simulink model "SensoryAttenuationTask"  (R2019b)
settings: Solver=ode4  StartTime=0.0  StopTime=inf  FixedStep=BKIN_STEP_TIME  RelTol=1e-3  EnableMultiTasking=on
StartFcn:
  |  warndlg('Dexterit-E models cannot run under simulation. Please compile your model and run it from within Dexterit-E.');set_param(bdroot,'SimulationCommand','stop')
model workspace (MAT data in the model file):
  BKIN_KINEMATIC_FRAME_SIZE = 400
  BKIN_STEP_TIME = 0.00025
  COLOR_2ND = 5
  COLOR_INIT = 4
  EDGE_COLOUR = 8
  EDGE_WIDTH = 9
  E_HAND_IN_START = 2
  E_MATCH_CHECK_ON = 8
  E_MATCH_END = 9
  E_MATCH_ON = 7
  E_MATCH_START = 8
  E_NO_EVENT = 0
  E_SLIDER_CHECK_ON = 4
  E_SLIDER_END = 5
  E_SLIDER_START = 10
  E_TEST_FORCE_ON = 3
  E_TIMED_OUT = 11
  E_TRIAL_END = 6
  E_TRIAL_START = 1
  HOLD_DELAY = 3
  LEFT_COL = 1
  LENGTH = 6
  LOAD_COL = 9
  LOAD_TIME = 4
  LOAD_X = 1
  LOAD_Y = 2
  MATCH_COL = 5
  MATCH_C_COL = 6
  MATCH_SCALING = 8
  MAX_START_TIME = 1
  RADIUS_VIS = 3
  RAMP_DURATION = 5
  RAMP_DURATION_EXAM = 6
  RIGHT_COL = 2
  SAFETY_DIST = 12
  SAFETY_SCALING = 13
  SLIDER_COL = 3
  SLIDER_C_COL = 4
  SLIDER_SCALING = 7
  SLOW_THRESH = 11
  TEXT = 10
  TEXT2_COL = 8
  TEXT_COL = 7
  TEXT_DISTH = 10
  TEXT_DISTV = 9
  TEXT_SIZE = 11
  WIDTH = 7
  WITHIN_DELAY = 2
  col_x = 1
  col_y = 2
undefined symbols (not defined in the file): slselsubs
libraries: Video x9, KINARM_general x5, General x3, KINARM_EP_loads x3
settings Model: ModifiedComment=chris -- Wed Feb 16 09:18:30 2005 -- Version 1.1384  ModifiedHistory=Feb 16/05 - Add error repeat, add offset ramp  ExtModeArmWhenConnect=off  ExtModeLogAll=off  OrderedModelArguments=off  Creator=Chris Grebeldinger  LastModifiedBy=User
settings SolverCC: AutoInsertRateTranBlk=on
settings DataIOCC: SaveFormat=Array  SignalLoggingSaveFormat=ModelDataLogs  SaveOutput=off  SaveTime=off  ReturnWorkspaceOutputs=off  SignalLoggingName=sigsOut
settings OptimizationCC: BlockReduction=off  BooleanDataType=off  OptimizeBlockIOStorage=off  BufferReuse=off  GlobalBufferReuse=off  ExpressionFolding=off  ExpressionDepthLimit=2147483647  LocalBlockOutputs=off  InitFltsAndDblsToZero=on  LifeSpan=inf  OptimizeDataStoreBuffers=off  BusAssignmentInplaceUpdate=off
settings DebuggingCC: SaveWithParameterizedLinksMsg=none  UnderspecifiedInitializationDetection=Classic  MergeDetectMultiDrivingBlocksExec=none  SignalResolutionControl=TryResolveAllWithWarning  MultiTaskDSMMsg=warning  FcnCallInpInsideContextMsg=warning  BusObjectLabelMismatch=none  StateNameClashWarn=warning  StrictBusMsg=ErrorOnBusTreatedAsVector  SFUnexpectedBacktrackingDiag=warning  SFNoUnconditionalDefaultTransitionDiag=warning  SFExecutionAtInitializationDiag=none  UnderSpecifiedDimensionMsg=warning  ArithmeticOperatorsInVariantConditions=warning
settings HardwareCC: ProdBitPerPointer=32  ProdBitPerSizeT=32  ProdBitPerPtrDiffT=32  ProdLargestAtomicFloat=None  ProdWordSize=32  ProdLongLongMode=on  ProdHWDeviceType=Generic->32-bit x86 compatible  TargetLongLongMode=on  TargetIntDivRoundTo=Zero  TargetEndianess=LittleEndian  TargetHWDeviceType=Generic->32-bit x86 compatible
settings ModelReferenceCC: PropagateSignalLabelsOutOfModel=off
settings SFSimCC: SimCustomHeaderCode="#include \"stdlib.h\""  SimUseLocalCustomCode=off  SimParseCustomCode=off  CustomCodeUndefinedFunction=UseInterfaceOnly
settings RTWCC: Description=Simulink Real-Time  SystemTargetFile=slrt.tlc  TemplateMakefile=slrt_default_tmf  RTWUseLocalCustomCode=off  CustomSourceCode="#include \"stdlib.h\""  CodeExecutionProfiling=on
settings CodeAppCC: MaxIdLength=63  StateflowObjectComments=on
settings SimulinkRealTimeCC: TargetFcnLib=ansi_tfl_tmw.mat  GeneratePreprocessorConditionals=Disable all  PreserveStateflowLocalDataDimensions=off
settings ConfigComp: CovMetricSettings=dw  CovHtmlReporting=on  CovSaveCumulativeToWorkspaceVar=on  CovSaveSingleToWorkspaceVar=on  CovExternalEMLEnable=off

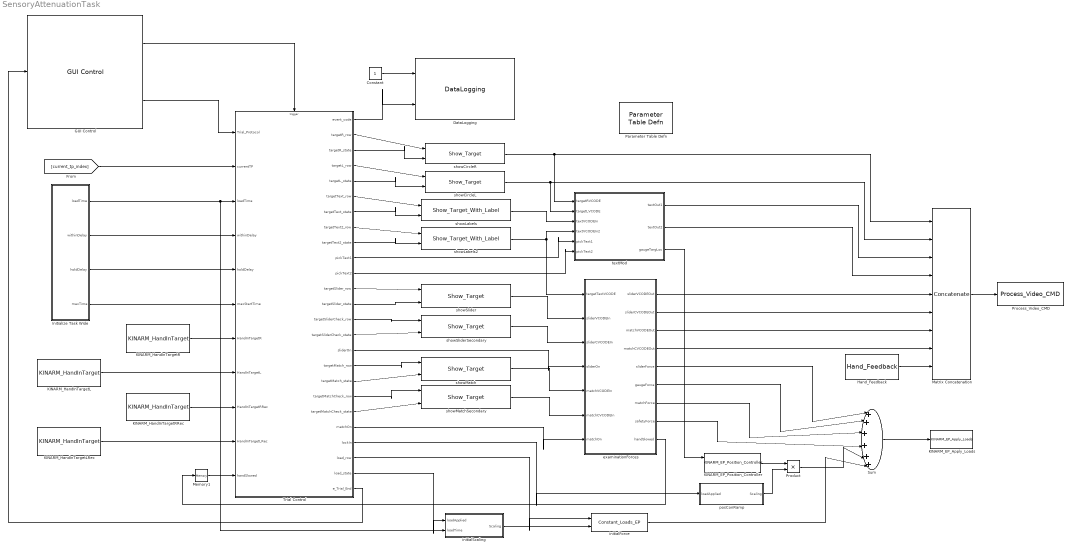
== system SensoryAttenuationTask ==
  Constant : Constant
  DataLogging : General/DataLogging  log_event_codes=on  log_analog_inputs=off  show_time_remaining=off  ecat_include=on
  GUI Control : General/GUI Control  task_version=1.0  show_repeat_trial_flag=off  use_custom_tp=off  target_type_str=Circle  Target_Type=1  XYcols=[1 2]  Vcols=3  Lcols=4  indices_padding=[0 0 0 0;0 0 0 0]  target_table_rows=64  load_table_rows=20  tp_table_rows=100
  Hand_Feedback : KINARM_general/Hand_Feedback  feedback_cntl_src=none
  Initialize Task Wide : Subsystem
  KINARM_EP_Apply_Loads : KINARM_EP_loads/KINARM_EP_Apply_Loads  up_duration=1500  down_duration=1500  max_force=15
  KINARM_EP_Position_Controller : KINARM_EP_loads/KINARM_EP_Position_Controller  use_dom_hand=off  inertias_for_FF=KINARM End Point robot  gain_choice=Standard Movement  sample_time=0.001
  KINARM_HandInTargetL : KINARM_general/KINARM_HandInTarget  use_dominant_hand=off  target_type=Circle  num_states=1  attribcol1=[RADIUS_VIS]  attribcol2=[0]  attribcol3=[0]  attribcol4=[0]  attribcol5=[0]
  KINARM_HandInTargetLRec : KINARM_general/KINARM_HandInTarget  use_dominant_hand=off  target_type=Rectangle  num_states=1  attribcol1=[WIDTH LENGTH 0]  attribcol2=[0 0 0]  attribcol3=[0 0 0]  attribcol4=[0 0 0]  attribcol5=[0 0 0]
  KINARM_HandInTargetR : KINARM_general/KINARM_HandInTarget  use_dominant_hand=on  target_type=Circle  num_states=1  attribcol1=[RADIUS_VIS]  attribcol2=[0]  attribcol3=[0]  attribcol4=[0]  attribcol5=[0]
  KINARM_HandInTargetRRec : KINARM_general/KINARM_HandInTarget  use_dominant_hand=on  target_type=Rectangle  num_states=1  attribcol1=[WIDTH LENGTH 0]  attribcol2=[0 0 0]  attribcol3=[0 0 0]  attribcol4=[0 0 0]  attribcol5=[0 0 0]
  Matrix Concatenation : Concatenate  NumInputs=9  Mode=Multidimensional array
  Memory1 : Memory
  Parameter Table Defn : General/Parameter Table Defn  ShowInLibBrowser=0
  Process_Video_CMD : Video/Process_Video_CMD  video_delay=50
  Product : Product
  Sum : Sum  Inputs=|++++++|
  Trial Control : Stateflow chart  TreatAsAtomicUnit=on
  examinationForces : Subsystem
  initialForce : KINARM_EP_loads/Constant_Loads_EP  use_dom_hand=on  loadcol=[1 2]  source=port  scaling=1  use_LH_coord=on
  initialScaling : Subsystem  mask(Perturbation){}
  posConRamp : Subsystem  mask(Perturbation){}
  showCircleL : Video/Show_Target  target_type=Circle  num_states=1  attribcol1=[COLOR_INIT 0 0 RADIUS_VIS]  attribcol2=[0 0 0 0]  attribcol3=[0 0 0 0]  attribcol4=[0 0 0 0]  attribcol5=[0 0 0 0]  stateindices_padding=[0 0 0 0 0 0 0;0 0 0 0 0 0 0;0 0 0 0 0 0 0;0 0 0 0 0 0 0;0 0 0 0 0 0 0]  source=dialog  opacity=100  target_display=Both subject and operator displays  num_col=4
  showCircleR : Video/Show_Target  target_type=Circle  num_states=1  attribcol1=[COLOR_INIT 0 0 RADIUS_VIS]  attribcol2=[0 0 0 0]  attribcol3=[0 0 0 0]  attribcol4=[0 0 0 0]  attribcol5=[0 0 0 0]  stateindices_padding=[0 0 0 0 0 0 0;0 0 0 0 0 0 0;0 0 0 0 0 0 0;0 0 0 0 0 0 0;0 0 0 0 0 0 0]  source=dialog  opacity=100  target_display=Both subject and operator displays  num_col=4
  showLabels : Video/Show_Target_With_Label  target_type=Circle  num_states=2  attribcol1=[0 0 0 0 TEXT COLOR_INIT TEXT_SIZE]  attribcol2=[0 0 0 0 TEXT COLOR_2ND RADIUS_VIS]  attribcol3=[0 0 0 0 0 0 0]  attribcol4=[0 0 0 0 0 0 0]  attribcol5=[0 0 0 0 0 0 0]  stateindices_padding=[0 0 0 0;0 0 0 0;0 0 0 0;0 0 0 0;0 0 0 0]  source=dialog  opacity=100  target_display=Both subject and operator displays
  showLabels2 : Video/Show_Target_With_Label  target_type=Circle  num_states=2  attribcol1=[0 0 0 0 TEXT COLOR_INIT TEXT_SIZE]  attribcol2=[0 0 0 0 TEXT COLOR_2ND RADIUS_VIS]  attribcol3=[0 0 0 0 0 0 0]  attribcol4=[0 0 0 0 0 0 0]  attribcol5=[0 0 0 0 0 0 0]  stateindices_padding=[0 0 0 0;0 0 0 0;0 0 0 0;0 0 0 0;0 0 0 0]  source=dialog  opacity=100  target_display=Both subject and operator displays
  showMatch : Video/Show_Target  target_type=Rectangle  num_states=1  attribcol1=[COLOR_INIT EDGE_COLOUR EDGE_WIDTH WIDTH LENGTH 0]  attribcol2=[0 0 0 0 0 0]  attribcol3=[0 0 0 0 0 0]  attribcol4=[0 0 0 0 0 0]  attribcol5=[0 0 0 0 0 0]  stateindices_padding=[0 0 0 0 0;0 0 0 0 0;0 0 0 0 0;0 0 0 0 0;0 0 0 0 0]  source=dialog  opacity=100  target_display=Both subject and operator displays  num_col=6
  showMatchSecondary : Video/Show_Target  target_type=Rectangle  num_states=2  attribcol1=[COLOR_INIT EDGE_COLOUR EDGE_WIDTH WIDTH LENGTH 0]  attribcol2=[COLOR_2ND EDGE_COLOUR EDGE_WIDTH WIDTH LENGTH 0]  attribcol3=[0 0 0 0 0 0]  attribcol4=[0 0 0 0 0 0]  attribcol5=[0 0 0 0 0 0]  stateindices_padding=[0 0 0 0 0;0 0 0 0 0;0 0 0 0 0;0 0 0 0 0;0 0 0 0 0]  source=dialog  opacity=100  target_display=Both subject and operator displays  num_col=6
  showSlider : Video/Show_Target  target_type=Rectangle  num_states=1  attribcol1=[COLOR_INIT EDGE_COLOUR EDGE_WIDTH WIDTH LENGTH 0]  attribcol2=[0 0 0 0 0 0]  attribcol3=[0 0 0 0 0 0]  attribcol4=[0 0 0 0 0 0]  attribcol5=[0 0 0 0 0 0]  stateindices_padding=[0 0 0 0 0;0 0 0 0 0;0 0 0 0 0;0 0 0 0 0;0 0 0 0 0]  source=dialog  opacity=100  target_display=Both subject and operator displays  num_col=6
  showSliderSecondary : Video/Show_Target  target_type=Rectangle  num_states=2  attribcol1=[COLOR_INIT COLOR_INIT EDGE_WIDTH WIDTH LENGTH 0]  attribcol2=[COLOR_2ND COLOR_2ND EDGE_WIDTH WIDTH LENGTH 0]  attribcol3=[0 0 0 0 0 0]  attribcol4=[0 0 0 0 0 0]  attribcol5=[0 0 0 0 0 0]  stateindices_padding=[0 0 0 0 0;0 0 0 0 0;0 0 0 0 0;0 0 0 0 0;0 0 0 0 0]  source=dialog  opacity=100  target_display=Both subject and operator displays  num_col=6
  textMod : Subsystem
  wires:
  Trial Control/25(e_Trial_End) -> GUI Control/1
  Trial Control/3(targetR_state) -> showCircleR/2
  Matrix Concatenation/1 -> Process_Video_CMD/1
  Trial Control/1(event_code) -> DataLogging/2
  showCircleR/1 -> textMod/1(targetRVCODE), Matrix Concatenation/1
  Hand_Feedback/1 -> Matrix Concatenation/9
  Constant/1 -> DataLogging/1
  GUI Control/2 -> Trial Control/1(Trial_Protocol)
  KINARM_HandInTargetR/1 -> Trial Control/7(HandInTargetR)
  KINARM_HandInTargetL/1 -> Trial Control/8(HandInTargetL)
  Initialize Task Wide/1(loadTime) -> initialScaling/2(loadTime), Trial Control/3(loadTime)
  Initialize Task Wide/2(withinDelay) -> Trial Control/4(withinDelay)
  Initialize Task Wide/4(maxTime) -> Trial Control/6(maxStartTime)
  [current_tp_index] -> Trial Control/2(currentTP)
  Trial Control/5(targetL_state) -> showCircleL/2
  Trial Control/14(targetSliderCheck_row) -> showSliderSecondary/1
  Trial Control/15(targetSliderCheck_state) -> showSliderSecondary/2
  Trial Control/24(load_state) -> initialScaling/1(loadApplied)
  initialScaling/1(Scaling) -> initialForce/2
  showSlider/1 -> examinationForces/2(sliderVCODEIn)
  showLabels/1 -> textMod/3(textVCODEIn)
  Trial Control/23(load_row) -> initialForce/1
  KINARM_HandInTargetRRec/1 -> Trial Control/9(HandInTargetRRec)
  KINARM_HandInTargetLRec/1 -> Trial Control/10(HandInTargetLRec)
  Trial Control/16(sliderOn) -> examinationForces/4(sliderOn)
  examinationForces/5(sliderForce) -> Sum/1
  initialForce/1 -> Sum/6
  Sum/1 -> KINARM_EP_Apply_Loads/1
  showMatch/1 -> examinationForces/5(matchVCODEIn)
  showMatchSecondary/1 -> examinationForces/6(matchCVCODEIn)
  Trial Control/19(targetMatchCheck_row) -> showMatchSecondary/1
  Trial Control/20(targetMatchCheck_state) -> showMatchSecondary/2
  examinationForces/7(matchForce) -> Sum/3
  examinationForces/6(gaugeForce) -> Sum/2
  Trial Control/21(matchOn) -> examinationForces/7(matchOn)
  Trial Control/10(pickText1) -> textMod/5(pickText1)
  Trial Control/11(pickText2) -> textMod/6(pickText2)
  textMod/2(textOut2) -> Matrix Concatenation/4
  textMod/1(textOut1) -> Matrix Concatenation/3
  Initialize Task Wide/3(holdDelay) -> Trial Control/5(holdDelay)
  Trial Control/12(targetSlider_row) -> showSlider/1
  Trial Control/17(targetMatch_row) -> showMatch/1
  Trial Control/18(targetMatch_state) -> showMatch/2
  Trial Control/13(targetSlider_state) -> showSlider/2
  Trial Control/2(targetR_row) -> showCircleR/1
  Trial Control/4(targetL_row) -> showCircleL/1
  showCircleL/1 -> textMod/2(targetLVCODE), Matrix Concatenation/2
  Trial Control/6(targetText_row) -> showLabels/1
  Trial Control/7(targetText_state) -> showLabels/2
  Trial Control/8(targetText2_row) -> showLabels2/1
  Trial Control/9(targetText2_state) -> showLabels2/2
  showLabels2/1 -> textMod/4(textVCODEIn2), examinationForces/1(targetTextVCODE)
  showSliderSecondary/1 -> examinationForces/3(sliderCVCODEIn)
  examinationForces/1(sliderVCODEOut) -> Matrix Concatenation/5
  examinationForces/2(sliderCVCODEOut) -> Matrix Concatenation/6
  examinationForces/3(matchVCODEOut) -> Matrix Concatenation/7
  GUI Control/1 -> Trial Control/Trigger
  Memory1/1 -> Trial Control/11(handSlowed)
  examinationForces/4(matchCVCODEOut) -> Matrix Concatenation/8
  textMod/3(gaugeTargLoc) -> KINARM_EP_Position_Controller/1
  KINARM_EP_Position_Controller/1 -> Product/1
  Product/1 -> Sum/5
  Trial Control/22(lockIn) -> posConRamp/1(loadApplied)
  posConRamp/1(Scaling) -> Product/2
  examinationForces/9(handSlowed) -> Memory1/1
  examinationForces/8(safetyForce) -> Sum/4

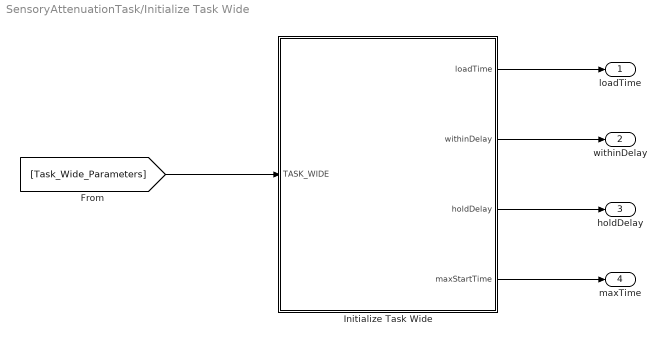
== system SensoryAttenuationTask/Initialize Task Wide ==
  Initialize Task Wide : MATLAB Function  TreatAsAtomicUnit=on
  loadTime : Outport
  withinDelay : Outport  Port=2
  holdDelay : Outport  Port=3
  maxTime : Outport  Port=4
  wires:
  [Task_Wide_Parameters] -> Initialize Task Wide/1(TASK_WIDE)
  Initialize Task Wide/1(loadTime) -> loadTime/1
  Initialize Task Wide/4(maxStartTime) -> maxTime/1
  Initialize Task Wide/2(withinDelay) -> withinDelay/1
  Initialize Task Wide/3(holdDelay) -> holdDelay/1

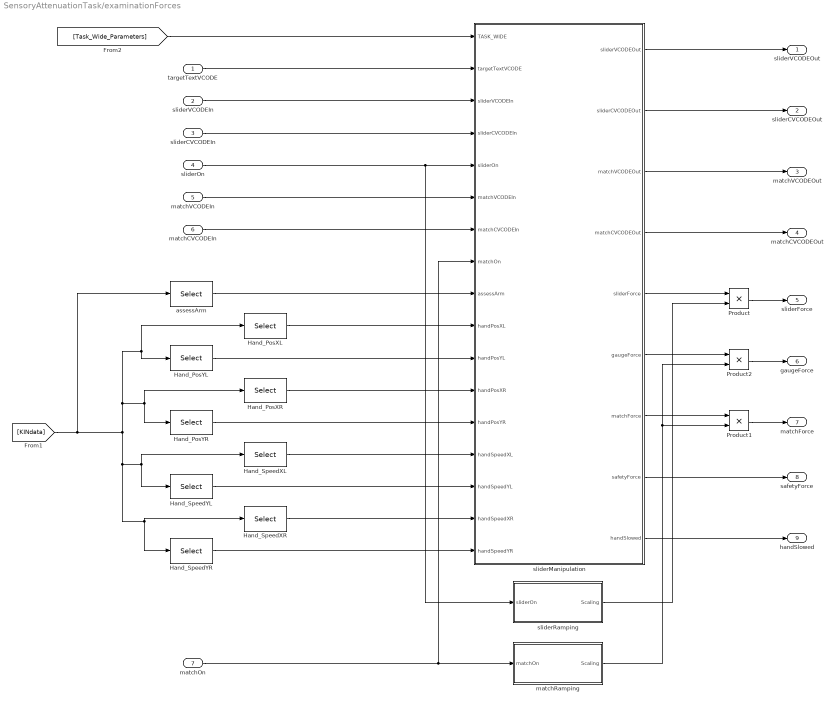
== system SensoryAttenuationTask/examinationForces ==
  targetTextVCODE : Inport
  sliderVCODEIn : Inport  Port=2
  sliderCVCODEIn : Inport  Port=3
  sliderOn : Inport  Port=4
  matchVCODEIn : Inport  Port=5
  matchCVCODEIn : Inport  Port=6
  matchOn : Inport  Port=7
  Hand_PosXL : Selector  NumberOfDimensions=2  InputPortWidth=3  IndexOptions=Index vector (dialog),Index vector (dialog)  Indices=[2],[23]  OutputSizes=slselsubs([(-2),(-2)],1),slselsubs([(-2),(-2)],2)
  Hand_PosXR : Selector  NumberOfDimensions=2  InputPortWidth=3  IndexOptions=Index vector (dialog),Index vector (dialog)  Indices=[1],[23]  OutputSizes=slselsubs([(-2),(-2)],1),slselsubs([(-2),(-2)],2)
  Hand_PosYL : Selector  NumberOfDimensions=2  InputPortWidth=3  IndexOptions=Index vector (dialog),Index vector (dialog)  Indices=[2],[24]  OutputSizes=slselsubs([(-2),(-2)],1),slselsubs([(-2),(-2)],2)
  Hand_PosYR : Selector  NumberOfDimensions=2  InputPortWidth=3  IndexOptions=Index vector (dialog),Index vector (dialog)  Indices=[1],[24]  OutputSizes=slselsubs([(-2),(-2)],1),slselsubs([(-2),(-2)],2)
  Hand_SpeedXL : Selector  NumberOfDimensions=2  InputPortWidth=3  IndexOptions=Index vector (dialog),Index vector (dialog)  Indices=[2],[25]  OutputSizes=slselsubs([(-2),(-2)],1),slselsubs([(-2),(-2)],2)
  Hand_SpeedXR : Selector  NumberOfDimensions=2  InputPortWidth=3  IndexOptions=Index vector (dialog),Index vector (dialog)  Indices=[1],[25]  OutputSizes=slselsubs([(-2),(-2)],1),slselsubs([(-2),(-2)],2)
  Hand_SpeedYL : Selector  NumberOfDimensions=2  InputPortWidth=3  IndexOptions=Index vector (dialog),Index vector (dialog)  Indices=[2],[26]  OutputSizes=slselsubs([(-2),(-2)],1),slselsubs([(-2),(-2)],2)
  Hand_SpeedYR : Selector  NumberOfDimensions=2  InputPortWidth=3  IndexOptions=Index vector (dialog),Index vector (dialog)  Indices=[1],[26]  OutputSizes=slselsubs([(-2),(-2)],1),slselsubs([(-2),(-2)],2)
  Product : Product
  Product1 : Product
  Product2 : Product
  assessArm : Selector  NumberOfDimensions=2  InputPortWidth=3  IndexOptions=Index vector (dialog),Index vector (dialog)  Indices=[3],[1]  OutputSizes=slselsubs([(-2),(-2)],1),slselsubs([(-2),(-2)],2)
  matchRamping : Subsystem  mask(Perturbation){}
  sliderManipulation : MATLAB Function  TreatAsAtomicUnit=on
  sliderRamping : Subsystem  mask(Perturbation){}
  sliderVCODEOut : Outport
  sliderCVCODEOut : Outport  Port=2
  matchVCODEOut : Outport  Port=3
  matchCVCODEOut : Outport  Port=4
  sliderForce : Outport  Port=5
  gaugeForce : Outport  Port=6
  matchForce : Outport  Port=7
  safetyForce : Outport  Port=8
  handSlowed : Outport  Port=9
  wires:
  sliderManipulation/2(sliderCVCODEOut) -> sliderCVCODEOut/1
  sliderManipulation/5(sliderForce) -> Product/1
  Hand_PosXR/1 -> sliderManipulation/12(handPosXR)
  Hand_PosXL/1 -> sliderManipulation/10(handPosXL)
  Hand_PosYL/1 -> sliderManipulation/11(handPosYL)
  Hand_PosYR/1 -> sliderManipulation/13(handPosYR)
  sliderCVCODEIn/1 -> sliderManipulation/4(sliderCVCODEIn)
  assessArm/1 -> sliderManipulation/9(assessArm)
  sliderVCODEIn/1 -> sliderManipulation/3(sliderVCODEIn)
  [Task_Wide_Parameters] -> sliderManipulation/1(TASK_WIDE)
  sliderOn/1 -> sliderManipulation/5(sliderOn), sliderRamping/1(sliderOn)
  sliderRamping/1(Scaling) -> Product/2
  Product/1 -> sliderForce/1
  matchOn/1 -> sliderManipulation/8(matchOn), matchRamping/1(matchOn)
  sliderManipulation/6(gaugeForce) -> Product2/1
  sliderManipulation/7(matchForce) -> Product1/1
  Product1/1 -> matchForce/1
  matchRamping/1(Scaling) -> Product2/2, Product1/2
  matchVCODEIn/1 -> sliderManipulation/6(matchVCODEIn)
  Product2/1 -> gaugeForce/1
  sliderManipulation/3(matchVCODEOut) -> matchVCODEOut/1
  matchCVCODEIn/1 -> sliderManipulation/7(matchCVCODEIn)
  sliderManipulation/1(sliderVCODEOut) -> sliderVCODEOut/1
  sliderManipulation/4(matchCVCODEOut) -> matchCVCODEOut/1
  [KINdata] -> assessArm/1, Hand_PosYR/1, Hand_PosXR/1, Hand_PosYL/1, Hand_PosXL/1, Hand_SpeedYR/1, Hand_SpeedXR/1, Hand_SpeedYL/1, Hand_SpeedXL/1
  Hand_SpeedXL/1 -> sliderManipulation/14(handSpeedXL)
  Hand_SpeedXR/1 -> sliderManipulation/16(handSpeedXR)
  Hand_SpeedYL/1 -> sliderManipulation/15(handSpeedYL)
  Hand_SpeedYR/1 -> sliderManipulation/17(handSpeedYR)
  sliderManipulation/9(handSlowed) -> handSlowed/1
  sliderManipulation/8(safetyForce) -> safetyForce/1
  targetTextVCODE/1 -> sliderManipulation/2(targetTextVCODE)

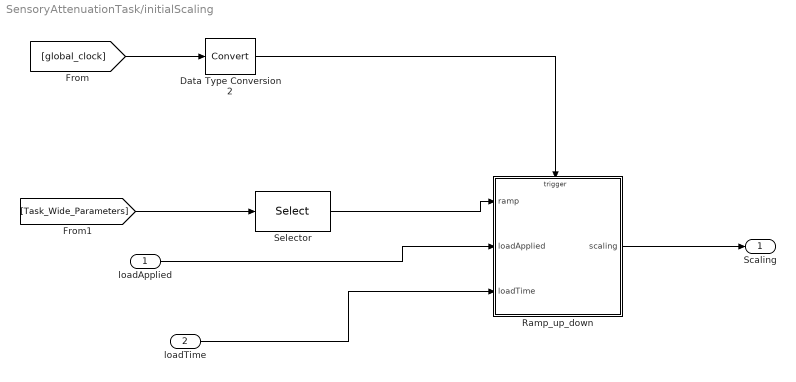
== system SensoryAttenuationTask/initialScaling ==
  loadApplied : Inport
  loadTime : Inport  Port=2
  Data Type Conversion2 : DataTypeConversion
  Ramp_up_down : Stateflow chart  TreatAsAtomicUnit=on
  Selector : Selector  NumberOfDimensions=2  InputPortWidth=3  IndexOptions=Index vector (dialog),Select all  Indices=[RAMP_DURATION],[3]  OutputSizes=slselsubs([(-2),(-2)],1),1
  Scaling : Outport
  wires:
  Ramp_up_down/1(scaling) -> Scaling/1
  [global_clock] -> Data Type Conversion2/1
  Data Type Conversion2/1 -> Ramp_up_down/Trigger
  [Task_Wide_Parameters] -> Selector/1
  Selector/1 -> Ramp_up_down/1(ramp)
  loadApplied/1 -> Ramp_up_down/2(loadApplied)
  loadTime/1 -> Ramp_up_down/3(loadTime)

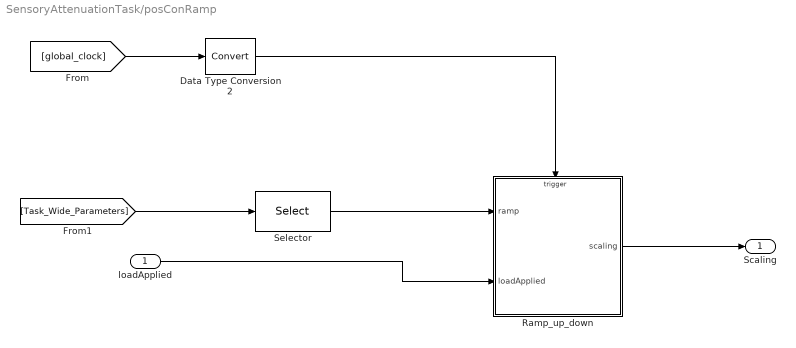
== system SensoryAttenuationTask/posConRamp ==
  loadApplied : Inport
  Data Type Conversion2 : DataTypeConversion
  Ramp_up_down : Stateflow chart  TreatAsAtomicUnit=on
  Selector : Selector  NumberOfDimensions=2  InputPortWidth=3  IndexOptions=Index vector (dialog),Select all  Indices=[RAMP_DURATION],[3]  OutputSizes=slselsubs([(-2),(-2)],1),1
  Scaling : Outport
  wires:
  Ramp_up_down/1(scaling) -> Scaling/1
  [global_clock] -> Data Type Conversion2/1
  Data Type Conversion2/1 -> Ramp_up_down/Trigger
  [Task_Wide_Parameters] -> Selector/1
  Selector/1 -> Ramp_up_down/1(ramp)
  loadApplied/1 -> Ramp_up_down/2(loadApplied)

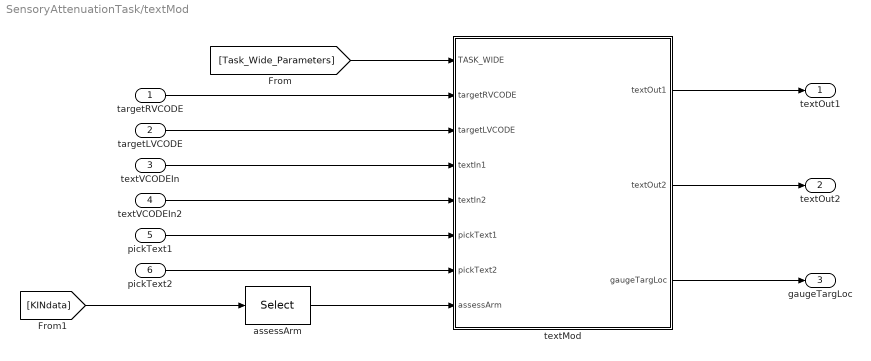
== system SensoryAttenuationTask/textMod ==
  targetRVCODE : Inport
  targetLVCODE : Inport  Port=2
  textVCODEIn : Inport  Port=3
  textVCODEIn2 : Inport  Port=4
  pickText1 : Inport  Port=5
  pickText2 : Inport  Port=6
  assessArm : Selector  NumberOfDimensions=2  InputPortWidth=3  IndexOptions=Index vector (dialog),Index vector (dialog)  Indices=[3],[1]  OutputSizes=slselsubs([(-2),(-2)],1),slselsubs([(-2),(-2)],2)
  textMod : MATLAB Function  TreatAsAtomicUnit=on
  textOut1 : Outport
  textOut2 : Outport  Port=2
  gaugeTargLoc : Outport  Port=3
  wires:
  textMod/1(textOut1) -> textOut1/1
  textMod/2(textOut2) -> textOut2/1
  textVCODEIn/1 -> textMod/4(textIn1)
  pickText1/1 -> textMod/6(pickText1)
  pickText2/1 -> textMod/7(pickText2)
  [Task_Wide_Parameters] -> textMod/1(TASK_WIDE)
  targetRVCODE/1 -> textMod/2(targetRVCODE)
  assessArm/1 -> textMod/8(assessArm)
  [KINdata] -> assessArm/1
  targetLVCODE/1 -> textMod/3(targetLVCODE)
  textVCODEIn2/1 -> textMod/5(textIn2)
  textMod/3(gaugeTargLoc) -> gaugeTargLoc/1

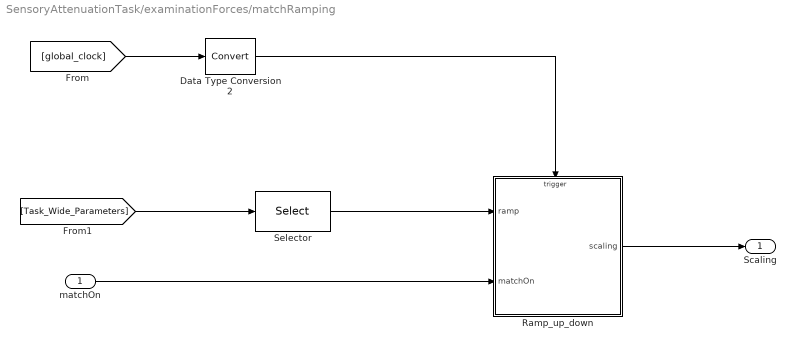
== system SensoryAttenuationTask/examinationForces/matchRamping ==
  matchOn : Inport
  Data Type Conversion2 : DataTypeConversion
  Ramp_up_down : Stateflow chart  TreatAsAtomicUnit=on
  Selector : Selector  NumberOfDimensions=2  InputPortWidth=3  IndexOptions=Index vector (dialog),Select all  Indices=[RAMP_DURATION_EXAM],[3]  OutputSizes=slselsubs([(-2),(-2)],1),1
  Scaling : Outport
  wires:
  Ramp_up_down/1(scaling) -> Scaling/1
  [global_clock] -> Data Type Conversion2/1
  Data Type Conversion2/1 -> Ramp_up_down/Trigger
  [Task_Wide_Parameters] -> Selector/1
  Selector/1 -> Ramp_up_down/1(ramp)
  matchOn/1 -> Ramp_up_down/2(matchOn)

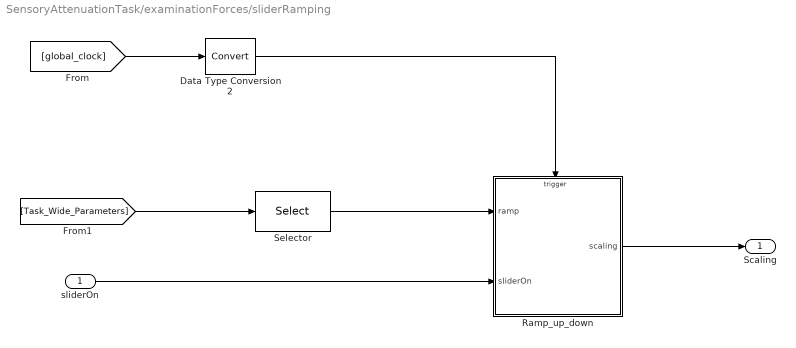
== system SensoryAttenuationTask/examinationForces/sliderRamping ==
  sliderOn : Inport
  Data Type Conversion2 : DataTypeConversion
  Ramp_up_down : Stateflow chart  TreatAsAtomicUnit=on
  Selector : Selector  NumberOfDimensions=2  InputPortWidth=3  IndexOptions=Index vector (dialog),Select all  Indices=[RAMP_DURATION_EXAM],[3]  OutputSizes=slselsubs([(-2),(-2)],1),1
  Scaling : Outport
  wires:
  Ramp_up_down/1(scaling) -> Scaling/1
  [global_clock] -> Data Type Conversion2/1
  Data Type Conversion2/1 -> Ramp_up_down/Trigger
  [Task_Wide_Parameters] -> Selector/1
  Selector/1 -> Ramp_up_down/1(ramp)
  sliderOn/1 -> Ramp_up_down/2(sliderOn)

== matlab function SensoryAttenuationTask/Initialize Task Wide/Initialize Task Wide ==
  data: TASK_WIDE input; loadTime output; withinDelay output; holdDelay output; maxStartTime output; MAX_START_TIME parameter; WITHIN_DELAY parameter; LOAD_TIME parameter; HOLD_DELAY parameter
function [loadTime, withinDelay, holdDelay, maxStartTime] = fcn(TASK_WIDE, MAX_START_TIME, WITHIN_DELAY, LOAD_TIME, HOLD_DELAY)
%initialize task wide parameters

loadTime = TASK_WIDE(LOAD_TIME); %time of the applied test load
withinDelay = TASK_WIDE(WITHIN_DELAY); %intertrial delay
holdDelay = TASK_WIDE(HOLD_DELAY); %time to hold hand steady for gauging
maxStartTime = TASK_WIDE(MAX_START_TIME); %time to initiate trial

== stateflow chart SensoryAttenuationTask/Trial Control ==
  state Initialiize/
    %Task looks at gauging an applied force using a slider
    %or applying a matching force to the hand
    %If TP is less than 4 the trial type is a slider trial and if greater than
    %3 than it is a match trial.
    % initialize the target rows
    targetL_row = Trial_Protocol(LEFT_COL);
    targetR_row = Trial_Protocol(RIGHT_COL);
    targetText_row = Trial_Protocol(TEXT_COL);
    targetText2_row = Trial_Protocol(TEXT2_COL);
    targetSlider_row = Trial_Protocol(SLIDER_COL);
    targetSliderCheck_row = Trial_Protocol(SLIDER_C_COL);
    targetMatch_row = Trial_Protocol(MATCH_COL);
    targetMatchCheck_row = Trial_Protocol(MATCH_C_COL);
  state MainTrial
    state showStartofForce/
      %begin the countdown for the
      %test force starting at 3
      entry:
      targetText_state = 1;
      targetText2_state = 1;
      pickText1 = 2;
      pickText2 = 1;
      targetSlider_state = 0;
      targetSliderCheck_state = 0;
      targetMatch_state = 0;
      targetMatchCheck_state = 0;
      targetR_state = 1;
      sliderOn = 0;
      matchOn = 0;
      lockIn = 1;
      event_code = E_TRIAL_START;
    state showStart/
      %show targets and texts
      entry:
      targetL_state = 1;
      targetR_state = 1;
      targetText_state = 1;
      pickText1 = 1;
      pickText2 = 0;
      lockIn = 0;
    state countdownAt2/
      %shows countdown at 2
      entry:
      pickText2 = 2;
    state countdownAt1/
      %shows countdown at 1
      entry:
      pickText2 = 3;
    state applyForce/
      %applies force
      entry:
      load_row = Trial_Protocol(LOAD_COL);
      load_state = 1;
      event_code = E_TEST_FORCE_ON;
    state loadStop/
      %preemptively stop force
      entry:
      load_state = 0;
    state checkForceMatch/
      %begin match force gauging
      entry:
      targetL_state = 0;
      targetR_state = 1;
      targetText2_state = 1;
      pickText1 = 3;
      pickText2 = 5;
      targetMatch_state = 1;
      targetMatchCheck_state = 1;
      event_code = E_MATCH_START;
      lockIn = 0;
    state checkForceSlider/
      %begin slider force gauging
      entry:
      targetL_state = 0;
      targetR_state = 1;
      targetText2_state = 1;
      pickText1 = 3;
      pickText2 = 4;
      targetSlider_state = 1;
      targetSliderCheck_state = 1;
      event_code = E_SLIDER_START;
      lockIn = 0;
    state timedOut/
      %check for slow start trials
      entry:
      event_code = E_TIMED_OUT;
    state checkMatch/
      %matching started
      entry:
      matchOn = 1;
      event_code = E_MATCH_CHECK_ON;
      targetMatchCheck_state = 1;
    state matchGauged/
      %change colour to indicate movement stop
      entry:
      targetMatchCheck_state = 2;
    state checkSlider/
      %slider started
      entry:
      sliderOn = 1;
      event_code = E_SLIDER_CHECK_ON;
      targetSliderCheck_state = 1;
    state sliderGauged/
      %change colour for movement stop
      entry:
      targetSliderCheck_state = 2;
    state EndOfMatch/
      % Turn off the targets
      entry:
      event_code = E_MATCH_END;
      matchOn = 0;
      targetMatchCheck_state = 0;
      targetMatch_state = 0;
    state EndOfSlider/
      % Turn off targets
      entry:
      event_code = E_SLIDER_END;
      sliderOn = 0;
      targetSliderCheck_state = 0;
      targetSlider_state = 0;
    showStart -> (junction 66) [order 1] : %check if both hands are in
        | [HandInTargetR(targetR_row) == 1]
    showStart -> (junction 66) [order 2] : [HandInTargetL(targetL_row) == 1]
    (junction 66) -> showStartofForce [order 3]
    (junction 66) -> showStart [order 2] : %check if either hand is out
        | [HandInTargetL(targetL_row) == 0]
    (junction 66) -> showStart [order 1] : [HandInTargetR(targetR_row) == 0]
    showStartofForce -> countdownAt2 : after(1000,msec)
    countdownAt1 -> applyForce : after(1000,msec)
    countdownAt2 -> countdownAt1 : after(1000,msec)
    showStart -> timedOut [order 3] : %check if participants didn't start the trial in time
        | after(maxStartTime, msec)
    applyForce -> loadStop : after(loadTime/2,msec)
    loadStop -> (junction 30) : after(loadTime/2,msec)
    (junction 30) -> checkForceMatch [order 1] : %if they are match trials
        | [currentTP > 3]
    (junction 30) -> checkForceSlider [order 2] : %if they are slider trials
        | [currentTP < 4]
    checkForceMatch -> checkMatch [order 2] : %check if hand is in match target
        | [HandInTargetLRec(targetMatch_row) == 1]
    checkForceMatch -> checkMatch [order 1] : %check if hand is in match target
        | [HandInTargetRRec(targetMatch_row) == 1]
    checkForceSlider -> checkSlider [order 1] : %check if hand is in slider target
        | [HandInTargetRRec(targetSlider_row) == 1]
    checkForceSlider -> checkSlider [order 2] : %check if hand is in slider target
        | [HandInTargetLRec(targetSlider_row) == 1]
    matchGauged -> checkMatch [order 2] : %hand started moving
        | [handSlowed == 0]
    timedOut -> (junction 99)
    sliderGauged -> checkSlider [order 2] : %hand started moving
        | [handSlowed == 0]
    checkMatch -> matchGauged : %hand stopped moving
        | [handSlowed == 1]
    matchGauged -> EndOfMatch [order 1] : %stayed still for long enough
        | after(holdDelay,msec)
    sliderGauged -> EndOfSlider [order 1] : %stayed still for long enough
        | after(holdDelay,msec)
    checkSlider -> sliderGauged : %hand stopped moving
        | [handSlowed == 1]
    EndOfMatch -> (junction 99)
    EndOfSlider -> (junction 99)
  state Inter_Trial_State/
    % Turn off all target
    entry:
    sliderOn = 0;
    matchOn = 0;
    pickText1 = 0;
    pickText2 = 0;
    targetSlider_state = 0;
    targetSliderCheck_state = 0;
    targetMatch_state = 0;
    targetMatchCheck_state = 0;
    targetText_state = 0;
    targetText2_state = 0;
    targetL_state = 0;
    targetR_state = 0;
    lockIn = 0;
    event_code = E_TRIAL_END;
    e_Trial_End;
  (default) -> Initialiize
  Initialiize -> showStart : %check if trial started
      | [currentTP > 0]
  Inter_Trial_State -> showStart : %after a certain period of time
      | after(withinDelay, msec)
  MainTrial -> Inter_Trial_State : e_ExitTrialNow/
      | {tickCount = 1;}
      | % e_ExitTrialNow event occurs if the
      | % Dex pause is pressed by the operator
  (junction 99) -> Inter_Trial_State : %after a certain period of time
      | after(withinDelay*2,msec)
  data: event_code output double [0..]; targetR_row output [1..32]; targetR_state output; targetL_row output; targetL_state output; targetText_row output; targetText_state output; targetText2_row output; targetText2_state output; pickText1 output; pickText2 output; targetSlider_row output; targetSlider_state output; targetSliderCheck_row output; targetSliderCheck_state output; sliderOn output; targetMatch_row output; targetMatch_state output; targetMatchCheck_row output; targetMatchCheck_state output; Trial_Protocol input double; currentTP input; loadTime input; withinDelay input; holdDelay input; maxStartTime input; HandInTargetR input; HandInTargetL input; matchOn output; lockIn output; load_row output; load_state output; HandInTargetRRec input; HandInTargetLRec input; tickCount local; handSlowed input double
  data targetR_row settings: description=index of the row currently being used in the TargetTable
  events: e_clk input RISING_EDGE_EVENT; e_ExitTrialNow input EITHER_EDGE_EVENT; e_Trial_End output EITHER_EDGE_EVENT

== matlab function SensoryAttenuationTask/examinationForces/sliderManipulation ==
  data: sliderVCODEOut output; TASK_WIDE input; targetTextVCODE input; sliderVCODEIn input; sliderCVCODEIn input; sliderOn input; matchVCODEIn input; matchCVCODEIn input; matchOn input; assessArm input; handPosXL input; handPosYL input; handPosXR input; handPosYR input; handSpeedXL input; handSpeedYL input; handSpeedXR input; handSpeedYR input; sliderCVCODEOut output; matchVCODEOut output; matchCVCODEOut output; sliderForce output; gaugeForce output; matchForce output; safetyForce output; handSlowed output; SLIDER_SCALING parameter; MATCH_SCALING parameter; SLOW_THRESH parameter; SAFETY_DIST parameter; SAFETY_SCALING parameter
function [sliderVCODEOut, sliderCVCODEOut, matchVCODEOut, matchCVCODEOut, sliderForce, gaugeForce, matchForce, safetyForce, handSlowed] = ...
fcn(TASK_WIDE, targetTextVCODE, sliderVCODEIn, sliderCVCODEIn,  sliderOn, matchVCODEIn, matchCVCODEIn, matchOn, assessArm, ...
handPosXL, handPosYL, handPosXR, handPosYR, handSpeedXL, handSpeedYL, handSpeedXR, handSpeedYR,...
SLIDER_SCALING, MATCH_SCALING, SLOW_THRESH, SAFETY_DIST, SAFETY_SCALING)
%This function applies test forces to a participant's arm to then gauge 
%using a slider or by matching the force with their other arm

%% initialize
sliderScaling = TASK_WIDE(SLIDER_SCALING); %scaling used to adjust gauging force
matchScaling = TASK_WIDE(MATCH_SCALING);
slowThresh = TASK_WIDE(SLOW_THRESH)*0.01; %speed threshold
safetyDist = TASK_WIDE(SAFETY_DIST)*0.01;
safetyScaling = TASK_WIDE(SAFETY_SCALING);

%get the dimesnions of the slider
sliderVCODEOut = sliderVCODEIn;
sliderCVCODEOut = sliderCVCODEIn;
sliderLoc = [sliderVCODEIn(3), sliderVCODEIn(4)]; %x y locations of the slider
sliderDim = [sliderVCODEIn(10), sliderVCODEIn(11)]; %width and length of the slider
sliderTop = sliderLoc(2)+sliderDim(2)/2; %top of the slider
sliderBot = sliderLoc(2)-sliderDim(2)/2; %bottom of the slider

%get the location of the match target
matchLoc = [matchCVCODEIn(3), matchCVCODEIn(4)]; %x y locations of the match box
matchVCODEOut = matchVCODEIn;
matchCVCODEOut = matchCVCODEIn;

%get the middle of the workspace
targetMidLoc = targetTextVCODE(3);

%% start gauging force on hands
if (assessArm == 2) %left arm assessed
    %set the hand position and speed to the right arm for gauging the force 
    %applied to the left arm
    handPosX = handPosXR;
    handPosY = handPosYR;
    handSpeedX = handSpeedXR;
    handSpeedY = handSpeedYR;
    
    %slider trials
    sliderForce = [0,0,-abs(handPosY-sliderCVCODEIn(4))*100*sliderScaling,0]; %apply force on left arm using right arm as gauge
    
    %match trials
    matchCVCODEOut(3) = matchLoc(1);
    if (handPosX < matchLoc(1)) %make sure to only apply force if hand is to the left of the match location
        matchForce = [0,0,(handPosX-matchLoc(1))*100*matchScaling,0]; %force on left arm from gauging right arm
        gaugeForce = [-(handPosX-matchLoc(1))*100,0,0,0]; %force on right arm to match test force
        if (matchOn == 1) %if the match gauge has begun
            matchCVCODEOut(3) = matchLoc(1)-abs(handPosX-matchLoc(1))/2; %base of rectangle representing amount of force
            matchCVCODEOut(10) = abs(handPosX-matchLoc(1)); %change length of rectangle based on amount of force
        end
    else %safety to not cause unwanted forces
        matchForce = [0,0,0,0];
        gaugeForce = [-abs(handPosX-matchLoc(1))*100*10,0,0,0];
    end
else %right arm assessed and same comments as above
    %set the hand position and speed to the left arm for gauging the force 
    %applied to the right arm
    handPosX = handPosXL;
    handPosY = handPosYL;
    handSpeedX = handSpeedXL;
    handSpeedY = handSpeedYL;
    
    %slider trials
    sliderForce = [abs(handPosY-sliderCVCODEIn(4))*100*sliderScaling,0,0,0];
    
    %match trials
    matchCVCODEOut(3) = matchLoc(1);
    if (handPosX > matchLoc(1))
        matchForce = [(handPosX-matchLoc(1))*100*matchScaling,0,0,0];
        gaugeForce = [0,0,-(handPosX-matchLoc(1))*100,0];
        if (matchOn == 1)
            matchCVCODEOut(3) = matchLoc(1)+abs(handPosX-matchLoc(1))/2;
            matchCVCODEOut(10) = abs(handPosX-matchLoc(1));
        end
    else
        matchForce = [0,0,0,0];
        gaugeForce = [0,0,abs(handPosX-matchLoc(1))*100*10,0];
    end
end

%% safety force
%barrier in the center of the workspace to make sure hands dont bump into
%each other after completing a match gauging trial
safetyForce = [0,0,0,0];
if (handPosXL > targetMidLoc-safetyDist) %check the left hand
    safetyForce = [0,0,-(handPosXL-(targetMidLoc-safetyDist))*100*safetyScaling,0];
end
if (handPosXR < targetMidLoc+safetyDist) %check the right hand
    safetyForce = [((targetMidLoc+safetyDist)-handPosXR)*100*safetyScaling,0,0,0];
end
if ((handPosXR < targetMidLoc+safetyDist) && (handPosXL > targetMidLoc-safetyDist)) %check if both hands in
    safetyForce = [((targetMidLoc+safetyDist)-handPosXR)*100*safetyScaling,0,-(handPosXL-(targetMidLoc-safetyDist))*100*safetyScaling,0];
end

%% slider visual
if (sliderOn == 1) %if slider is on, set a maximum and minimum limit for the visual to not go out of bounds
    sliderCVCODEOut(4) = handPosY;
    if (handPosY > sliderTop) %if the hand is above the top boundary
        handPosY = sliderTop;
    end
    if (handPosY < sliderBot) %if the hand is below the bottom boundary
        handPosY = sliderBot;
    end
end

%% check for slowed hand
%get a measure of the participants hand speed to check if they moved slower
%than a threshold
handSpeed = hypot(handSpeedX, handSpeedY);
if (handSpeed < slowThresh) %if the handspeed is lower than the threshold
    handSlowed = 1;
else
    handSlowed = 0;
end

forceCheck = [abs(handPosY-sliderLoc(2)-sliderDim(2)/2)*100];
handLoc = [handPosY sliderLoc(2) sliderDim(2)];

== stateflow chart SensoryAttenuationTask/examinationForces/sliderRamping/Ramp_up_down ==
  state peak/
    entry:
    scaling=1;
  state RampingUp/
    %sigmoidal ramping taken from Ethan Heming and
    %modified by Kayne
    entry:
    tick=0;
    CurrScale=scaling;
    b=ramp/4; % Center at Middle;
    c=ramp/20; % Define Rise Rate;
    during:
    tick++;
    scaling = (1-CurrScale)/(1+exp(-1*(tick-b)/c))+CurrScale;
  state RampingDown/
    entry:
    tick=0;
    CurrScale=scaling;
    b=ramp/4; % Center at Middle;
    c=ramp/20; % Define Drop Rate;
    during:
    tick++;
    scaling = CurrScale*(1-1/(1+exp(-1*(tick-b)/c)));
  state minimum/
    entry:
    scaling=0;
  RampingUp -> peak : after(ramp, e_clk)
  peak -> RampingDown : %after load time
      | [sliderOn == 0]
  RampingDown -> minimum : after(ramp, e_clk)
  minimum -> RampingUp : %check if hand is in target and
      | %trial has a forcefield
      | [sliderOn == 1]
  (default) -> minimum
  data: ramp input double; scaling output double; tick local double; c local double; b local double; CurrScale local double; sliderOn input double
  events: e_clk input RISING_EDGE_EVENT

== stateflow chart SensoryAttenuationTask/examinationForces/matchRamping/Ramp_up_down ==
  state peak/
    entry:
    scaling=1;
  state RampingUp/
    %sigmoidal ramping taken from Ethan Heming and
    %modified by Kayne
    entry:
    tick=0;
    CurrScale=scaling;
    b=ramp/4; % Center at Middle;
    c=ramp/20; % Define Rise Rate;
    during:
    tick++;
    scaling = (1-CurrScale)/(1+exp(-1*(tick-b)/c))+CurrScale;
  state RampingDown/
    entry:
    tick=0;
    CurrScale=scaling;
    b=ramp/4; % Center at Middle;
    c=ramp/20; % Define Drop Rate;
    during:
    tick++;
    scaling = CurrScale*(1-1/(1+exp(-1*(tick-b)/c)));
  state minimum/
    entry:
    scaling=0;
  RampingUp -> peak : after(ramp, e_clk)
  peak -> RampingDown : %after load time
      | [matchOn != 1]
  RampingDown -> minimum : after(ramp, e_clk)
  minimum -> RampingUp : %check if hand is in target and
      | %trial has a forcefield
      | [matchOn == 1]
  (default) -> minimum
  data: ramp input double; scaling output double; tick local double; c local double; b local double; CurrScale local double; matchOn input double
  events: e_clk input RISING_EDGE_EVENT

== matlab function SensoryAttenuationTask/textMod/textMod ==
  data: TASK_WIDE input; targetRVCODE input; targetLVCODE input; textOut1 output; textOut2 output; textIn1 input; textIn2 input; pickText1 input; pickText2 input; assessArm input; TEXT_DISTH parameter; TEXT_DISTV parameter; gaugeTargLoc output
function [textOut1, textOut2, gaugeTargLoc] = fcn(TASK_WIDE, targetRVCODE, targetLVCODE, textIn1, textIn2, pickText1, pickText2, assessArm, TEXT_DISTH, TEXT_DISTV)
%This function modifies the text shown to participants at the top of the
%screen and below the gauging hand.

%% initialize
textDistV = TASK_WIDE(TEXT_DISTV)/100; %adjustment of the offset for the supplemental text
textDistH = TASK_WIDE(TEXT_DISTH)/100;

%get the assessed arm
if (assessArm == 1)
    armPick = 'right hand';
else
    armPick = 'left hand';
end
gaugeTargX = targetLVCODE(3); %x position of the gauged target
gaugeTargY = targetLVCODE(4); %y position of the gauged target

%modify text at the stop of the screen
textOut1 = textIn1;
if (pickText1 == 1)
    str1 = ['Place your hands in the circles to start the force'];
elseif (pickText1 == 2)
    str1 = ['Resist the force on your ', armPick, ' starting in:'];
elseif (pickText1 == 3)
    str1 = ['Estimate the force by moving your ', armPick];
else
    str1 = ' ';
end
textOut1(1,15:(length(str1)+14))=uint16(str1);  %str in letters

%text of target that supplements textOut1
textOut2 = textIn2;
if (pickText2 == 1) %modify the text below the text at the top of the screen
    textOut2(4) = textIn2(4)-textDistV;
    str2 = '3...';
elseif (pickText2 == 2)
    textOut2(4) = textIn2(4)-textDistV;
    str2 = '2..';
elseif (pickText2 == 3)
    textOut2(4) = textIn2(4)-textDistV;
    str2 = '1.';
elseif (pickText2 == 4) %modify text shown below the gauging hand
    textOut2(3) = gaugeTargX;
    textOut2(4) = gaugeTargY-textDistV;
    str2 = 'Hold still to lock in your estimate';
elseif (pickText2 == 5)
    textOut2(3) = gaugeTargX;
    textOut2(4) = gaugeTargY-textDistV;
    str2 = 'Hold still to lock in your estimate';
else
    str2 = ' ';
end
textOut2(1,15:(length(str2)+14))=uint16(str2);

textLoc = [textIn2(3) textIn2(4) textOut2(3) textOut2(4) textDistV textDistH];
gaugeTargLoc = [gaugeTargX gaugeTargY];

== stateflow chart SensoryAttenuationTask/posConRamp/Ramp_up_down ==
  state peak/
    entry:
    scaling=1;
  state RampingUp/
    %sigmoidal ramping taken from Ethan Heming and
    %modified by Kayne
    entry:
    tick=0;
    CurrScale=scaling;
    b=ramp/4; % Center at Middle;
    c=ramp/20; % Define Rise Rate;
    during:
    tick++;
    scaling = (1-CurrScale)/(1+exp(-1*(tick-b)/c))+CurrScale;
  state RampingDown/
    entry:
    tick=0;
    CurrScale=scaling;
    b=ramp/4; % Center at Middle;
    c=ramp/20; % Define Drop Rate;
    during:
    tick++;
    scaling = CurrScale*(1-1/(1+exp(-1*(tick-b)/c)));
  state minimum/
    entry:
    scaling=0;
  RampingUp -> peak : after(ramp, e_clk)
  peak -> RampingDown : %after load time
      | [loadApplied == 0]
  RampingDown -> minimum : after(ramp, e_clk)
  minimum -> RampingUp : %check if hand is in target and
      | %trial has a forcefield
      | [loadApplied == 1]
  (default) -> minimum
  data: ramp input double; scaling output double; tick local double; c local double; b local double; CurrScale local double; loadApplied input double
  events: e_clk input RISING_EDGE_EVENT

== stateflow chart SensoryAttenuationTask/initialScaling/Ramp_up_down ==
  state peak/
    entry:
    scaling=1;
  state RampingUp/
    %sigmoidal ramping taken from Ethan Heming and
    %modified by Kayne
    entry:
    tick=0;
    CurrScale=scaling;
    b=ramp/4; % Center at Middle;
    c=ramp/20; % Define Rise Rate;
    during:
    tick++;
    scaling = (1-CurrScale)/(1+exp(-1*(tick-b)/c))+CurrScale;
  state RampingDown/
    entry:
    tick=0;
    CurrScale=scaling;
    b=ramp/4; % Center at Middle;
    c=ramp/20; % Define Drop Rate;
    during:
    tick++;
    scaling = CurrScale*(1-1/(1+exp(-1*(tick-b)/c)));
  state minimum/
    entry:
    scaling=0;
  RampingUp -> peak : after(ramp, e_clk)
  peak -> RampingDown : %after load time
      | after(loadTime-ramp*2,msec)
  RampingDown -> minimum : after(ramp, e_clk)
  minimum -> RampingUp : %check if hand is in target and
      | %trial has a forcefield
      | [loadApplied == 1]
  (default) -> minimum
  data: ramp input double; scaling output double; tick local double; c local double; b local double; CurrScale local double; loadApplied input double; loadTime input double
  events: e_clk input RISING_EDGE_EVENT
